simulink library "ddm"  (R2021b)
settings: Solver=VariableStepAuto  StartTime=0.0  StopTime=10.0  RelTol=1e-3
undefined symbols (not defined in the file): ADDM_FrTMTqDev_X_Nm, ADDM_RrTMTqDev_X_Nm, ENUM_ADASACCSTA_ERROR, ENUM_ADASACCSTA_OFF, ENUM_ADASACCSTA_STANDBY, ENUM_ALLOWMOV_ALLOWREADY, ENUM_APS, ENUM_BRKSTA_ERROR, ENUM_BRKSTA_OFF, ENUM_BRKSTA_ON, ENUM_BRKSW_INVALID, ENUM_BRKSW_OFF, ENUM_BRKSW_ON, ENUM_CHGPREACTERRSTA_OBCPRE, ENUM_DCDCFAULTSTA_ANYFAULTLV1, ENUM_DCDCFAULTSTA_ANYFAULTLV2, ENUM_DRIVETRAIN_AWD, ENUM_DRIVETRAIN_FWD, ENUM_DRIVETRAIN_RWD, ENUM_EDUDRTSTA_NORMAL, ENUM_EPBERROR_FAILED, ENUM_EPBSTA_APPLIED, ENUM_EPBSTA_RELEASED, ENUM_ESCAPSSta_APSUNAVAILABLE, ENUM_GEARACTUALPOSN_INVALID, ENUM_GEARACTUALPOSN_P, ENUM_HVBATTREADYPRE_READY, ENUM_HWRESETSTA_HWRESETING, ENUM_MCUWARN_LV0, ENUM_MCUWARN_LV1, ENUM_MCUWARN_LV2, ENUM_MCUWARN_LV3, ENUM_MCUWARN_NOERROR, ENUM_OBCFAULTSTA_ANYFAULT, ENUM_PAS_R2F2, ENUM_PDFAULT_BATTPDFAIL, ENUM_PDFAULT_DCDCDISABLE, ENUM_PDFAULT_MCUDISABLE, ENUM_PDFAULT_MCUDISCHRG, ENUM_POWERSTA_OFF, ENUM_POWERSTA_ON, ENUM_POWERSTA_READY, ENUM_POWERSTA_STANDBY, ENUM_PRESSINDI_LOW, ENUM_PUFAULT_BATTUPFAIL, ENUM_PUFAULT_DCDCENABLEFAIL, ENUM_PUFAULT_PRECHRGCHKFAIL, ENUM_PUFAULT_SAFETYCHKFAIL, ENUM_PWRSTASW_OFF, ENUM_PWRSTASW_OFFA, ENUM_PWRSTASW_OFFCHVCHRG, ENUM_PWRSTASW_OFFCLVCHRG, ENUM_PWRSTASW_ON, ENUM_PWRSTASW_ONHVCHRG, ENUM_PWRSTASW_READY, ENUM_PWRSTASW_STANDBY, ENUM_RAPSErrWarnSta_NORMAL, ENUM_RAPSErrWarnSta_RAPSERRLV1, ENUM_SHIFTCOMMAND_P, ENUM_SHIFTERERRSTA_PBUTTONFAILURE ... (+471)
libraries: hcu_lib x540, simulink x3
(part 6 of 26)

== system ddm/DDM/DDM/TPM ==
  note: SensorFail
  note: WheelTmpHigh
  note: PressureLow
  note: Batwarn
  task_time_s : Inport
  VPMM_PowerSta_enum : Inport  Port=2
  DTC_clear_request : Inport  Port=3
  VDDM_ClearZevDTCcmd_flg : Inport  Port=4
  VTPM_LFBatwarn_flg : Inport  Port=5
  VTPM_RFBatwarn_flg : Inport  Port=6
  VTPM_LRBatwarn_flg : Inport  Port=7
  VTPM_RRBatwarn_flg : Inport  Port=8
  VTPM_LFPressIndi_enum : Inport  Port=9
  VTPM_RFPressIndi_enum : Inport  Port=10
  VTPM_LRPressIndi_enum : Inport  Port=11
  VTPM_RRPressIndi_enum : Inport  Port=12
  VTPM_LFWheelTmpIndi_flg : Inport  Port=13
  VTPM_RFWheelTmpIndi_flg : Inport  Port=14
  VTPM_LRWheelTmpIndi_flg : Inport  Port=15
  VTPM_RRWheelTmpIndi_flg : Inport  Port=16
  VTPM_LFSensorFail_flg : Inport  Port=17
  VTPM_RFSensorFail_flg : Inport  Port=18
  VTPM_LRSensorFail_flg : Inport  Port=19
  VTPM_RRSensorFail_flg : Inport  Port=20
  LFBatwarn : Subsystem
  LFPressureLow : Subsystem
  LFSensorfail : Subsystem
  LFWheelTmpHigh : Subsystem
  LRBatwarn : Subsystem
  LRPressureLow : Subsystem
  LRSensorfail : Subsystem
  LRWheelTmpHigh : Subsystem
  RFBatwarn : Subsystem
  RFPressureLow : Subsystem
  RFSensorfail : Subsystem
  RFWheelTmpHigh : Subsystem
  RRBatwarn : Subsystem
  RRPressureLow : Subsystem
  RRSensorfail : Subsystem
  RRWheelTmpHigh : Subsystem
  VDDM_LFBatwarnDTC_raw32 : Outport
  VDDM_RFBatwarnDTC_raw32 : Outport  Port=2
  VDDM_LRBatwarnDTC_raw32 : Outport  Port=3
  VDDM_RRBatwarnDTC_raw32 : Outport  Port=4
  VDDM_LFPressIndiDTC_raw32 : Outport  Port=5
  VDDM_RFPressIndiDTC_raw32 : Outport  Port=6
  VDDM_LRPressIndiDTC_raw32 : Outport  Port=7
  VDDM_RRPressIndiDTC_raw32 : Outport  Port=8
  VDDM_LFWheelTmpHighDTC_raw32 : Outport  Port=9
  VDDM_RFWheelTmpHighDTC_raw32 : Outport  Port=10
  VDDM_LRWheelTmpHighDTC_raw32 : Outport  Port=11
  VDDM_RRWheelTmpHighDTC_raw32 : Outport  Port=12
  VDDM_LFSensorFailDTC_raw32 : Outport  Port=13
  VDDM_RFSensorFailDTC_raw32 : Outport  Port=14
  VDDM_LRSensorFailDTC_raw32 : Outport  Port=15
  VDDM_RRSensorFailDTC_raw32 : Outport  Port=16
  wires:
  VPMM_PowerSta_enum/1 -> [VPMM_PowerSta_enum]
  DTC_clear_request/1 -> [DTC_clear_request]
  task_time_s/1 -> [task_time_s]
  [VPMM_PowerSta_enum] -> LFBatwarn/2(VPMM_PowerSta_enum)
  [task_time_s] -> LFBatwarn/1(task_time_s)
  [DTC_clear_request] -> LFBatwarn/3(DTC_clear_request)
  VTPM_LFBatwarn_flg/1 -> LFBatwarn/4(VTPM_LFBatwarn_flg)
  LFBatwarn/1(VDDM_LFBatwarnDTC_raw32) -> VDDM_LFBatwarnDTC_raw32/1
  [task_time_s] -> RFBatwarn/1(task_time_s)
  [VPMM_PowerSta_enum] -> RFBatwarn/2(VPMM_PowerSta_enum)
  [DTC_clear_request] -> RFBatwarn/3(DTC_clear_request)
  VTPM_RFBatwarn_flg/1 -> RFBatwarn/4(VTPM_RFBatwarn_flg)
  RFBatwarn/1(VDDM_RFBatwarnDTC_raw32) -> VDDM_RFBatwarnDTC_raw32/1
  [task_time_s] -> LRBatwarn/1(task_time_s)
  [VPMM_PowerSta_enum] -> LRBatwarn/2(VPMM_PowerSta_enum)
  [DTC_clear_request] -> LRBatwarn/3(DTC_clear_request)
  VTPM_LRBatwarn_flg/1 -> LRBatwarn/4(VTPM_LRBatwarn_flg)
  LRBatwarn/1(VDDM_LRBatwarnDTC_raw32) -> VDDM_LRBatwarnDTC_raw32/1
  RRBatwarn/1(VDDM_RRBatwarnDTC_raw32) -> VDDM_RRBatwarnDTC_raw32/1
  [task_time_s] -> RRBatwarn/1(task_time_s)
  [VPMM_PowerSta_enum] -> RRBatwarn/2(VPMM_PowerSta_enum)
  [DTC_clear_request] -> RRBatwarn/3(DTC_clear_request)
  VTPM_RRBatwarn_flg/1 -> RRBatwarn/4(VTPM_RRBatwarn_flg)
  [task_time_s] -> LFPressureLow/1(task_time_s)
  [VPMM_PowerSta_enum] -> LFPressureLow/2(VPMM_PowerSta_enum)
  [VDDM_ClearZevDTCcmd_flg] -> LFPressureLow/3(DTC_clear_request)
  [task_time_s] -> RFPressureLow/1(task_time_s)
  [VPMM_PowerSta_enum] -> RFPressureLow/2(VPMM_PowerSta_enum)
  [VDDM_ClearZevDTCcmd_flg] -> RFPressureLow/3(DTC_clear_request)
  [VDDM_ClearZevDTCcmd_flg] -> LRPressureLow/3(DTC_clear_request)
  [VPMM_PowerSta_enum] -> LRPressureLow/2(VPMM_PowerSta_enum)
  [task_time_s] -> LRPressureLow/1(task_time_s)
  [task_time_s] -> RRPressureLow/1(task_time_s)
  [VPMM_PowerSta_enum] -> RRPressureLow/2(VPMM_PowerSta_enum)
  [VDDM_ClearZevDTCcmd_flg] -> RRPressureLow/3(DTC_clear_request)
  LFPressureLow/1(VDDM_LFPressIndiDTC_raw32) -> VDDM_LFPressIndiDTC_raw32/1
  RFPressureLow/1(VDDM_RFPressIndiDTC_raw32) -> VDDM_RFPressIndiDTC_raw32/1
  LRPressureLow/1(VDDM_LRPressIndiDTC_raw32) -> VDDM_LRPressIndiDTC_raw32/1
  RRPressureLow/1(VDDM_RRPressIndiDTC_raw32) -> VDDM_RRPressIndiDTC_raw32/1
  VTPM_LFPressIndi_enum/1 -> LFPressureLow/4(VTPM_LFPressIndi_enum)
  VTPM_RFPressIndi_enum/1 -> RFPressureLow/4(VTPM_RFPressIndi_enum)
  VTPM_LRPressIndi_enum/1 -> LRPressureLow/4(VTPM_LRPressIndi_enum)
  VTPM_RRPressIndi_enum/1 -> RRPressureLow/4(VTPM_RRPressIndi_enum)
  [task_time_s] -> LFWheelTmpHigh/1(task_time_s)
  [VPMM_PowerSta_enum] -> LFWheelTmpHigh/2(VPMM_PowerSta_enum)
  [DTC_clear_request] -> LFWheelTmpHigh/3(DTC_clear_request)
  [task_time_s] -> RFWheelTmpHigh/1(task_time_s)
  [VPMM_PowerSta_enum] -> RFWheelTmpHigh/2(VPMM_PowerSta_enum)
  [DTC_clear_request] -> RFWheelTmpHigh/3(DTC_clear_request)
  [task_time_s] -> LRWheelTmpHigh/1(task_time_s)
  [VPMM_PowerSta_enum] -> LRWheelTmpHigh/2(VPMM_PowerSta_enum)
  [DTC_clear_request] -> LRWheelTmpHigh/3(DTC_clear_request)
  [task_time_s] -> RRWheelTmpHigh/1(task_time_s)
  [VPMM_PowerSta_enum] -> RRWheelTmpHigh/2(VPMM_PowerSta_enum)
  [DTC_clear_request] -> RRWheelTmpHigh/3(DTC_clear_request)
  VTPM_LFWheelTmpIndi_flg/1 -> LFWheelTmpHigh/4(VTPM_LFWheelTmpHigh_flg)
  VTPM_RFWheelTmpIndi_flg/1 -> RFWheelTmpHigh/4(VTPM_RFWheelTmpHigh_flg)
  VTPM_LRWheelTmpIndi_flg/1 -> LRWheelTmpHigh/4(VTPM_LRWheelTmpHigh_flg)
  VTPM_RRWheelTmpIndi_flg/1 -> RRWheelTmpHigh/4(VTPM_RRWheelTmpHigh_flg)
  LFWheelTmpHigh/1(VDDM_LFWheelTmpHighDTC_raw32) -> VDDM_LFWheelTmpHighDTC_raw32/1
  RFWheelTmpHigh/1(VDDM_RFWheelTmpHighDTC_raw32) -> VDDM_RFWheelTmpHighDTC_raw32/1
  LRWheelTmpHigh/1(VDDM_LRWheelTmpHighDTC_raw32) -> VDDM_LRWheelTmpHighDTC_raw32/1
  RRWheelTmpHigh/1(VDDM_RRWheelTmpHighDTC_raw32) -> VDDM_RRWheelTmpHighDTC_raw32/1
  [task_time_s] -> LFSensorfail/1(task_time_s)
  [VPMM_PowerSta_enum] -> LFSensorfail/2(VPMM_PowerSta_enum)
  [VDDM_ClearZevDTCcmd_flg] -> LFSensorfail/3(DTC_clear_request)
  [task_time_s] -> RFSensorfail/1(task_time_s)
  [VPMM_PowerSta_enum] -> RFSensorfail/2(VPMM_PowerSta_enum)
  [VDDM_ClearZevDTCcmd_flg] -> RFSensorfail/3(DTC_clear_request)
  [task_time_s] -> LRSensorfail/1(task_time_s)
  [VPMM_PowerSta_enum] -> LRSensorfail/2(VPMM_PowerSta_enum)
  [VDDM_ClearZevDTCcmd_flg] -> LRSensorfail/3(DTC_clear_request)
  [task_time_s] -> RRSensorfail/1(task_time_s)
  [VPMM_PowerSta_enum] -> RRSensorfail/2(VPMM_PowerSta_enum)
  [VDDM_ClearZevDTCcmd_flg] -> RRSensorfail/3(DTC_clear_request)
  VTPM_LFSensorFail_flg/1 -> LFSensorfail/4(VTPM_LFSensorFail_flg)
  VTPM_RFSensorFail_flg/1 -> RFSensorfail/4(VTPM_RFSensorFail_flg)
  VTPM_LRSensorFail_flg/1 -> LRSensorfail/4(VTPM_LRSensorFail_flg)
  VTPM_RRSensorFail_flg/1 -> RRSensorfail/4(VTPM_RRSensorFail_flg)
  LFSensorfail/1(VDDM_LFSensorFailDTC_raw32) -> VDDM_LFSensorFailDTC_raw32/1
  RFSensorfail/1(VDDM_RFSensorFailDTC_raw32) -> VDDM_RFSensorFailDTC_raw32/1
  LRSensorfail/1(VDDM_LRSensorFailDTC_raw32) -> VDDM_LRSensorFailDTC_raw32/1
  RRSensorfail/1(VDDM_RRSensorFailDTC_raw32) -> VDDM_RRSensorFailDTC_raw32/1
  VDDM_ClearZevDTCcmd_flg/1 -> [VDDM_ClearZevDTCcmd_flg]

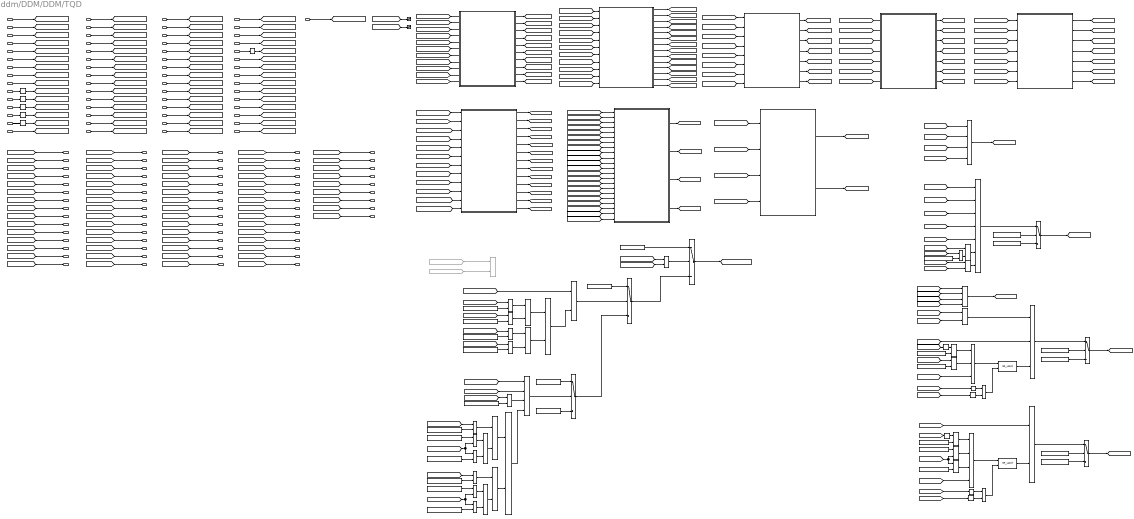
== system ddm/DDM/DDM/TQD ==
  note: VDDM_EPB1Err_flg
  note: Shifeter Error lamp Signal
  note: Three-electrical warning
  note: Warning lamp Signal
  note: RAPS Signal error
  VPMM_SysPwrSta_enum : Inport
  VINP_AccelPedal1Vol_V : Inport  Port=2
  VINP_AccelPedal2Vol_V : Inport  Port=3
  VDHP_EAPS12RangeSta_enum : Inport  Port=4
  VDHP_EAPCRBAD_flg : Inport  Port=5
  task_time_s : Inport  Port=6
  DTC_clear_request : Inport  Port=7
  No_CAN3_BUS_OFF : Inport  Port=8
  No_CAN1_BUS_OFF : Inport  Port=9
  VDDM_CANMsgValidMCUF1_flg : Inport  Port=10
  VDDM_CANMsgValidMCUR1_flg : Inport  Port=11
  VINP_CANMsgValidShifter1_flg : Inport  Port=12
  VINP_CANMsgValidESC1_flg : Inport  Port=13
  VINP_CANMsgValidESC5_flg : Inport  Port=14
  VDDM_MCUF1RCErr_flg : Inport  Port=15
  VDDM_MCUF1CSErr_flg : Inport  Port=16
  VDDM_MCUR1RCErr_flg : Inport  Port=17
  VDDM_MCUR1CSErr_flg : Inport  Port=18
  VDDM_Shifter1RCErr_flg : Inport  Port=19
  VDDM_Shifter1CSErr_flg : Inport  Port=20
  VDDM_ESC1RCErr_flg : Inport  Port=21
  VDDM_ESC1CSErr_flg : Inport  Port=22
  VDDM_ESC5RCErr_flg : Inport  Port=23
  VDDM_ESC5CSErr_flg : Inport  Port=24
  VINP_FrEDUDrtSta_flg : Inport  Port=25
  VINP_VehSpeed_kph : Inport  Port=26
  VINP_FrEDURealTMTq_Nm : Inport  Port=27
  VTQR_FrTMTqReq_Nm : Inport  Port=28
  VINP_RrEDUDrtSta_flg : Inport  Port=29
  VINP_RrEDURealTMTq_Nm : Inport  Port=30
  VTQR_RrTMTqReq_Nm : Inport  Port=31
  VINP_MCUWarnF_enum : Inport  Port=32
  VINP_MCUWarnR_enum : Inport  Port=33
  VINP_Pedal1Ref5V_V : Inport  Port=34
  VINP_Pedal2Ref5V_V : Inport  Port=35
  VINP_HVBattSOC_pct : Inport  Port=36
  VDDM_AuxBattVolV_V : Inport  Port=37
  VTQD_ActParkRequest_flg : Inport  Port=38
  VINP_EPBSta_enum : Inport  Port=39
  VINP_ShifterHandleCmd_enum : Inport  Port=40
  VINP_BMSWarn4_flg : Inport  Port=41
  VINP_BMSWarn5_flg : Inport  Port=42
  VINP_BMSWarn6_flg : Inport  Port=43
  VINP_BMSWarn7_flg : Inport  Port=44
  VINP_BMSWarn8_flg : Inport  Port=45
  VINP_DCDCFaultSta_enum : Inport  Port=46
  VPMM_DrivetrainSelect_enum : Inport  Port=47
  VTQD_GearActualPosn_enum : Inport  Port=48
  VINP_EPBErrSta_enum : Inport  Port=49
  VINP_CANMsgValidEPB1_flg : Inport  Port=50
  VDDM_EPB1RCErr_flg : Inport  Port=51
  VDDM_EPB1CSErr_flg : Inport  Port=52
  VDHP_EAPS1BAD_flg : Inport  Port=53
  VDHP_EAPS2BAD_flg : Inport  Port=54
  VDDM_C3BMS1LCCFS_flg : Inport  Port=55
  VDDM_VCURAPSErrLv2_flg : Inport  Port=56
  VVMC_APSActive_flg : Inport  Port=57
  VDDM_ClearZevDTCcmd_flg : Inport  Port=58
  VDDM_LimpHomeAct_flg : Inport  Port=59
  VTQR_FrTqZeroTrans_enum : Inport  Port=60
  VTQR_RrTqZeroTrans_enum : Inport  Port=61
  APS_DDM : Subsystem
  Constant : Constant  Value=KDDM_SysErrShifterErrSW_flg
  Constant1 : Constant  Value=ENUM_DRIVETRAIN_FWD
  Constant10 : Constant  Value=ENUM_MCUWARN_LV3
  Constant11 : Constant  Value=ENUM_VEHMALFUNLV_3RD
  Constant12 : Constant  Value=ENUM_VEHMALFUNLV_4TH
  Constant{13..14,18..19,88} (5 alike) : Constant  Value=ENUM_GEARACTUALPOSN_P
  Constant15 : Constant  Value=ENUM_VEHMALFUNLV_2ND
  Constant16 : Constant  Value=ENUM_VEHMALFUNLV_NORMAL
  Constant17 : Constant  Value=ENUM_DCDCFAULTSTA_ANYFAULTLV2
  Constant2 : Constant  Value=ENUM_MCUWARN_LV1
  Constant20 : Constant  Value=ENUM_GEARACTUALPOSN_INVALID
  Constant21 : Constant  Value=FALSE
  Constant22 : Constant  Value=KDDM_EPBErrPopupSW_flg
  Constant23 : Constant  Value=FALSE
  Constant24 : Constant  Value=KDDM_EPBErrPopupSW_flg
  Constant25 : Constant  Value=FALSE
  Constant3 : Constant  Value=ENUM_MCUWARN_LV2
  Constant4 : Constant  Value=ENUM_DRIVETRAIN_RWD
  Constant5 : Constant  Value=ENUM_MCUWARN_LV1
  Constant6 : Constant  Value=ENUM_MCUWARN_LV2
  Constant7 : Constant  Value=ENUM_DRIVETRAIN_FWD
  Constant8 : Constant  Value=ENUM_DRIVETRAIN_RWD
  Constant9 : Constant  Value=ENUM_MCUWARN_LV3
  Delay{,1..3} (4 alike) : Delay  DelayLength=1
  EPB : Subsystem
  ESC1_DDM : Subsystem
  ESC5_DDM : Subsystem
  Equal{,1,5,8,11,15..16} (7 alike) : RelationalOperator  Operator=~=  OutDataTypeStr=boolean  RndMeth=Simplest
  Equal{2..4,6..7,9..10,12..14} (10 alike) : RelationalOperator  Operator===  OutDataTypeStr=boolean  RndMeth=Simplest
  From112 : From  Commented=on  GotoTag=VDDM_MCUNR1NoComCFS_flg
  From176 : From  Commented=on  GotoTag=VDDM_C3BMS1LCCFS_flg
  Logical Operator{,1,3..5,8,12..13} (8 alike) : Logic  Operator=NOT  AllPortsSameDT=off  OutDataTypeStr=boolean
  Logical Operator10 : Logic  Inputs=4  AllPortsSameDT=off  OutDataTypeStr=boolean
  Logical Operator11 : Logic  AllPortsSameDT=off  OutDataTypeStr=boolean
  Logical Operator14 : Logic  Operator=OR  AllPortsSameDT=off  OutDataTypeStr=boolean
  Logical Operator15 : Logic  Operator=OR  AllPortsSameDT=off  OutDataTypeStr=boolean
  Logical Operator2 : Logic  AllPortsSameDT=off  OutDataTypeStr=boolean
  Logical Operator6 : Logic  AllPortsSameDT=off  OutDataTypeStr=boolean
  Logical Operator7 : Logic  Inputs=3  AllPortsSameDT=off  OutDataTypeStr=boolean
  Logical Operator9 : Logic  Operator=OR  Inputs=4  AllPortsSameDT=off  OutDataTypeStr=boolean
  MCU1_DDM : Subsystem
  MCU_DDM : Subsystem
  OR : Logic  Operator=OR  Inputs=4  AllPortsSameDT=off  OutDataTypeStr=boolean
  OR1 : Logic  Operator=OR  Inputs=7  AllPortsSameDT=off  OutDataTypeStr=boolean
  OR{4,6..7,9..10,12,14} (7 alike) : Logic  Operator=OR  AllPortsSameDT=off  OutDataTypeStr=boolean
  OR{5,8,11,13} (4 alike) : Logic  AllPortsSameDT=off  OutDataTypeStr=boolean
  OR15 : Logic  Commented=on  Operator=OR  AllPortsSameDT=off  OutDataTypeStr=boolean
  OR2 : Logic  Operator=OR  Inputs=3  AllPortsSameDT=off  OutDataTypeStr=boolean
  OR3 : Logic  Operator=OR  Inputs=4  AllPortsSameDT=off  OutDataTypeStr=boolean
  Regen_fail_DDM : Subsystem
  SR_Latch1 : hcu_lib/Basic_Blocks/SR_Latch
  SR_Latch2 : hcu_lib/Basic_Blocks/SR_Latch
  Shifter1_DDM : Subsystem
  Switch : Switch  Criteria=u2 > Threshold
  Switch1 : Switch  Criteria=u2 ~= 0
  Switch2 : Switch  Criteria=u2 ~= 0
  Switch3 : Switch  Criteria=u2 > Threshold
  Switch4 : Switch  Criteria=u2 > Threshold
  Switch6 : Switch  Criteria=u2 ~= 0
  Terminator : Terminator
  Terminator1 : Terminator
  VDDM_APS1SigOoRDTC_raw32 : Outport
  VDDM_APS2SigOoRDTC_raw32 : Outport  Port=2
  VDDM_APSCorrErrDTC_raw32 : Outport  Port=3
  VDDM_MCUF1NoComDTC_raw32 : Outport  Port=4
  VDDM_MCUR1NoComDTC_raw32 : Outport  Port=5
  VDDM_Shifter1NoComDTC_raw32 : Outport  Port=6
  VDDM_ESC1NoComDTC_raw32 : Outport  Port=7
  VDDM_ESC5NoComDTC_raw32 : Outport  Port=8
  VDDM_MCUF1RCErrDTC_raw32 : Outport  Port=9
  VDDM_MCUR1RCErrDTC_raw32 : Outport  Port=10
  VDDM_MCUF1CSErrDTC_raw32 : Outport  Port=11
  VDDM_MCUR1CSErrDTC_raw32 : Outport  Port=12
  VDDM_Shifter1RCErrDTC_raw32 : Outport  Port=13
  VDDM_Shifter1CSErrDTC_raw32 : Outport  Port=14
  VDDM_ESC1RCErrDTC_raw32 : Outport  Port=15
  VDDM_ESC1CSErrDTC_raw32 : Outport  Port=16
  VDDM_ESC5RCErrDTC_raw32 : Outport  Port=17
  VDDM_ESC5CSErrDTC_raw32 : Outport  Port=18
  VDDM_FrMCUTqErrDTC_raw32 : Outport  Port=19
  VDDM_RrMCUTqErrDTC_raw32 : Outport  Port=20
  VDDM_MCUF1NoComCFS_flg : Outport  Port=21
  VDDM_MCUF1RCErrCFS_flg : Outport  Port=22
  VDDM_MCUF1CSErrCFS_flg : Outport  Port=23
  VDDM_MCUR1NoComCFS_flg : Outport  Port=24
  VDDM_MCUR1RCErrCFS_flg : Outport  Port=25
  VDDM_MCUR1CSErrCFS_flg : Outport  Port=26
  VDDM_ESC1NoComCFS_flg : Outport  Port=27
  VDDM_ESC1RCErrCFS_flg : Outport  Port=28
  VDDM_ESC1CSErrCFS_flg : Outport  Port=29
  VDDM_ESC5NoComCFS_flg : Outport  Port=30
  VDDM_ESC5RCErrCFS_flg : Outport  Port=31
  VDDM_ESC5CSErrCFS_flg : Outport  Port=32
  VDDM_5vAPS1OoRDTC_raw32 : Outport  Port=33
  VDDM_5vAPS2OoRDTC_raw32 : Outport  Port=34
  VDDM_EDriveSysErrTQD_flg : Outport  Port=35
  VDDM_EDriveSysErrShifterErr_flg : Outport  Port=36
  VDDM_EngagePFail_flg : Outport  Port=37
  VDDM_VehMalfunLevelTmp_enum : Outport  Port=38
  VDDM_EPBLockTODTC_raw32 : Outport  Port=39
  VDDM_EPBUnlockTODTC_raw32 : Outport  Port=40
  VDDM_EPB1NoComDTC_raw32 : Outport  Port=41
  VDDM_EPB1RCErrDTC_raw32 : Outport  Port=42
  VDDM_EPB1CSErrDTC_raw32 : Outport  Port=43
  VDDM_EPBSigErrDTC_raw32 : Outport  Port=44
  VDDM_5vAPS1OoRCFS_flg : Outport  Port=45
  VDDM_5vAPS2OoRCFS_flg : Outport  Port=46
  VDDM_APS1SigOoRCFS_flg : Outport  Port=47
  VDDM_APS2SigOoRCFS_flg : Outport  Port=48
  VDDM_APSCorrErrCFS_flg : Outport  Port=49
  VDDM_Shifter1NoComCFS_flg : Outport  Port=50
  VDDM_Shifter1RCErrCFS_flg : Outport  Port=51
  VDDM_Shifter1CSErrCFS_flg : Outport  Port=52
  VDDM_EPBSigErrCFS_flg : Outport  Port=53
  VDDM_EPB1NoComCFS_flg : Outport  Port=54
  VDDM_EPB1RCErrCFS_flg : Outport  Port=55
  VDDM_EPB1CSErrCFS_flg : Outport  Port=56
  VDDM_EPBLockTOCFS_flg : Outport  Port=57
  VDDM_EPBUnlockTOCFS_flg : Outport  Port=58
  VDDM_FrMCUTqErrCFS_flg : Outport  Port=59
  VDDM_RrMCUTqErrCFS_flg : Outport  Port=60
  VDDM_DisengagePFail_flg : Outport  Port=61
  VDDM_Shifter1Err_flg : Outport  Port=62
  VDDM_EPB1Err_flg : Outport  Port=63
  VDDM_ESC5Err_flg : Outport  Port=64
  VDDM_ESC1Err_flg : Outport  Port=65
  VDDM_RegenErrDTC_raw32 : Outport  Port=66
  VDDM_RegenErrCFS_flg : Outport  Port=67
  VDDM_MCUF1Err_flg : Outport  Port=68
  VDDM_MCUR1Err_flg : Outport  Port=69
  wires:
  VINP_ShifterHandleCmd_enum/1 -> [VINP_ShifterHandleCmd_enum]
  VINP_EPBSta_enum/1 -> [VINP_EPBSta_enum]
  VTQD_ActParkRequest_flg/1 -> [VTQD_ActParkRequest_flg]
  VDDM_AuxBattVolV_V/1 -> [VDDM_AuxBattVolV_V]
  VINP_HVBattSOC_pct/1 -> [VINP_HVBattSOC_pct]
  [VINP_Pedal2Ref5V_V] -> APS_DDM/7(VINP_Pedal2Ref5V_V)
  [VINP_Pedal1Ref5V_V] -> APS_DDM/6(VINP_Pedal1Ref5V_V)
  VINP_Pedal2Ref5V_V/1 -> [VINP_Pedal2Ref5V_V]
  VINP_Pedal1Ref5V_V/1 -> [VINP_Pedal1Ref5V_V]
  [VDDM_MCUR1RCErrCFS_flg] -> MCU_DDM/12(VDDM_MCUR1RCErrCFS_flg)
  [VDDM_MCUF1RCErrCFS_flg] -> MCU_DDM/5(VDDM_MCUF1RCErrCFS_flg)
  [VDDM_MCUF1CSErrCFS_flg] -> MCU_DDM/6(VDDM_MCUF1CSErrCFS_flg)
  [No_CAN3_BUS_OFF] -> MCU_DDM/3(No_CAN3_BUS_OFF)
  [VINP_MCUWarnF_enum] -> MCU_DDM/17(VINP_MCUWarnF_enum)
  [VINP_RrEDUDrtSta_flg] -> MCU_DDM/14(VINP_RrEDUDrtSta_flg)
  [VDDM_MCUR1CSErrCFS_flg] -> MCU_DDM/13(VDDM_MCUR1CSErrCFS_flg)
  [VPMM_SysPwrSta_enum] -> MCU_DDM/2(VPMM_SysPwrSta_enum)
  [VDDM_MCUF1NoComCFS_flg] -> MCU_DDM/4(VDDM_MCUF1NoComCFS_flg)
  [VTQR_FrTMTqReq_Nm] -> MCU_DDM/10(VTQR_FrTMTqReq_Nm)
  [task_time_s] -> MCU_DDM/1(task_time_s)
  [VTQR_RrTMTqReq_Nm] -> MCU_DDM/16(VTQR_RrTMTqReq_Nm)
  [VINP_FrEDUDrtSta_flg] -> MCU_DDM/8(VINP_FrEDUDrtSta_flg)
  [VINP_FrEDURealTMTq_Nm] -> MCU_DDM/9(VINP_FrEDURealTMTq_Nm)
  [VINP_RrEDURealTMTq_Nm] -> MCU_DDM/15(VINP_RrEDURealTMTq_Nm)
  [VDDM_ClearZevDTCcmd_flg] -> MCU_DDM/19(DTC_clear_request)
  [VDDM_MCUR1NoComCFS_flg] -> MCU_DDM/11(VDDM_MCUR1NoComCFS_flg)
  [VINP_MCUWarnR_enum] -> MCU_DDM/18(VINP_MCUWarnR_enum)
  [VINP_VehSpeed_kph] -> MCU_DDM/7(VINP_VehSpeed_kph)
  [VDDM_MCUF1RCErrCFS_flg] -> VDDM_MCUF1RCErrCFS_flg/1
  [VDDM_MCUR1RCErrCFS_flg] -> VDDM_MCUR1RCErrCFS_flg/1
  [VDDM_MCUR1NoComCFS_flg] -> VDDM_MCUR1NoComCFS_flg/1
  [VDDM_MCUF1CSErrCFS_flg] -> VDDM_MCUF1CSErrCFS_flg/1
  [VDDM_MCUR1CSErrCFS_flg] -> VDDM_MCUR1CSErrCFS_flg/1
  [VDDM_MCUF1NoComCFS_flg] -> VDDM_MCUF1NoComCFS_flg/1
  MCU1_DDM/11(VDDM_MCUR1RCErrCFS_flg) -> [VDDM_MCUR1RCErrCFS_flg]
  MCU1_DDM/7(VDDM_MCUF1NoComCFS_flg) -> [VDDM_MCUF1NoComCFS_flg]
  MCU1_DDM/10(VDDM_MCUR1NoComCFS_flg) -> [VDDM_MCUR1NoComCFS_flg]
  MCU1_DDM/9(VDDM_MCUF1CSErrCFS_flg) -> [VDDM_MCUF1CSErrCFS_flg]
  MCU1_DDM/8(VDDM_MCUF1RCErrCFS_flg) -> [VDDM_MCUF1RCErrCFS_flg]
  MCU1_DDM/12(VDDM_MCUR1CSErrCFS_flg) -> [VDDM_MCUR1CSErrCFS_flg]
  VINP_MCUWarnR_enum/1 -> [VINP_MCUWarnR_enum]
  VINP_MCUWarnF_enum/1 -> [VINP_MCUWarnF_enum]
  VINP_VehSpeed_kph/1 -> [VINP_VehSpeed_kph]
  VINP_RrEDUDrtSta_flg/1 -> [VINP_RrEDUDrtSta_flg]
  VTQR_FrTMTqReq_Nm/1 -> [VTQR_FrTMTqReq_Nm]
  VINP_FrEDURealTMTq_Nm/1 -> [VINP_FrEDURealTMTq_Nm]
  VTQR_RrTMTqReq_Nm/1 -> [VTQR_RrTMTqReq_Nm]
  VINP_FrEDUDrtSta_flg/1 -> [VINP_FrEDUDrtSta_flg]
  VINP_RrEDURealTMTq_Nm/1 -> [VINP_RrEDURealTMTq_Nm]
  VDDM_ESC5RCErr_flg/1 -> [VDDM_ESC5RCErr_flg]
  VDDM_ESC5CSErr_flg/1 -> [VDDM_ESC5CSErr_flg]
  [VDDM_ESC5CSErr_flg] -> ESC5_DDM/6(VDDM_ESC5CSErr_flg)
  [VDDM_ESC5RCErr_flg] -> ESC5_DDM/5(VDDM_ESC5RCErr_flg)
  VDDM_ESC1RCErr_flg/1 -> [VDDM_ESC1RCErr_flg]
  VDDM_ESC1CSErr_flg/1 -> [VDDM_ESC1CSErr_flg]
  VDDM_Shifter1CSErr_flg/1 -> [VDDM_Shifter1CSErr_flg]
  VDDM_Shifter1RCErr_flg/1 -> [VDDM_Shifter1RCErr_flg]
  VDDM_MCUF1RCErr_flg/1 -> [VDDM_MCUF1RCErr_flg]
  VDDM_MCUF1CSErr_flg/1 -> [VDDM_MCUF1CSErr_flg]
  VDDM_MCUR1CSErr_flg/1 -> [VDDM_MCUR1CSErr_flg]
  VDDM_MCUR1RCErr_flg/1 -> [VDDM_MCUR1RCErr_flg]
  [VDDM_Shifter1CSErr_flg] -> Shifter1_DDM/6(VDDM_Shifter1CSErr_flg)
  [VDDM_Shifter1RCErr_flg] -> Shifter1_DDM/5(VDDM_Shifter1RCErr_flg)
  [VDDM_MCUR1CSErr_flg] -> MCU1_DDM/9(VDDM_MCUR1CSErr_flg)
  [VDDM_MCUR1RCErr_flg] -> MCU1_DDM/8(VDDM_MCUR1RCErr_flg)
  [VDDM_MCUF1CSErr_flg] -> MCU1_DDM/7(VDDM_MCUF1CSErr_flg)
  [VDDM_MCUF1RCErr_flg] -> MCU1_DDM/6(VDDM_MCUF1RCErr_flg)
  Logical Operator5/1 -> [VDDM_MCUF1NoCom_flg]
  Logical Operator4/1 -> [VDDM_MCUR1NoCom_flg]
  Logical Operator3/1 -> [VDDM_Shifter1NoCom_flg]
  Logical Operator1/1 -> [VDDM_ESC1NoCom_flg]
  Logical Operator/1 -> [VDDM_ESC5NoCom_flg]
  VINP_CANMsgValidESC5_flg/1 -> Logical Operator/1
  VINP_CANMsgValidESC1_flg/1 -> Logical Operator1/1
  VINP_CANMsgValidShifter1_flg/1 -> Logical Operator3/1
  VDDM_CANMsgValidMCUR1_flg/1 -> Logical Operator4/1
  VDDM_CANMsgValidMCUF1_flg/1 -> Logical Operator5/1
  No_CAN1_BUS_OFF/1 -> [No_CAN1_BUS_OFF]
  No_CAN3_BUS_OFF/1 -> [No_CAN3_BUS_OFF]
  [VDDM_ClearZevDTCcmd_flg] -> ESC5_DDM/7(DTC_clear_request)
  [VDDM_ESC5NoCom_flg] -> ESC5_DDM/4(VDDM_ESC5NoCom_flg)
  [No_CAN1_BUS_OFF] -> ESC5_DDM/3(No_CAN1_BUS_OFF)
  [VPMM_SysPwrSta_enum] -> ESC5_DDM/2(VPMM_SysPwrSta_enum)
  [task_time_s] -> ESC5_DDM/1(task_time_s)
  [No_CAN1_BUS_OFF] -> ESC1_DDM/3(No_CAN1_BUS_OFF)
  [VPMM_SysPwrSta_enum] -> ESC1_DDM/2(VPMM_SysPwrSta_enum)
  [task_time_s] -> ESC1_DDM/1(task_time_s)
  [VDDM_ClearZevDTCcmd_flg] -> Shifter1_DDM/7(DTC_clear_request)
  [VDDM_Shifter1NoCom_flg] -> Shifter1_DDM/4(VDDM_Shifter1NoCom_flg)
  [No_CAN3_BUS_OFF] -> Shifter1_DDM/3(No_CAN3_BUS_OFF)
  [VPMM_SysPwrSta_enum] -> Shifter1_DDM/2(VPMM_SysPwrSta_enum)
  [VDDM_ClearZevDTCcmd_flg] -> MCU1_DDM/10(DTC_clear_request)
  [VDDM_MCUR1NoCom_flg] -> MCU1_DDM/5(VDDM_MCUR1NoCom_flg)
  [VDDM_MCUF1NoCom_flg] -> MCU1_DDM/4(VDDM_MCUF1NoCom_flg)
  [No_CAN3_BUS_OFF] -> MCU1_DDM/3(No_CAN3_BUS_OFF)
  [VPMM_SysPwrSta_enum] -> MCU1_DDM/2(VPMM_SysPwrSta_enum)
  [task_time_s] -> Shifter1_DDM/1(task_time_s)
  [task_time_s] -> MCU1_DDM/1(task_time_s)
  DTC_clear_request/1 -> [DTC_clear_request]
  task_time_s/1 -> [task_time_s]
  [VDHP_EAPS12RangeSta_enum] -> APS_DDM/4(VDHP_EAPS12RangeSta_enum)
  [VINP_AccelPedal2Vol_V] -> APS_DDM/3(VINP_AccelPedal2Vol_V)
  [VINP_AccelPedal1Vol_V] -> APS_DDM/2(VINP_AccelPedal1Vol_V)
  [VPMM_SysPwrSta_enum] -> APS_DDM/1(VPMM_SysPwrSta_enum)
  [VDHP_EAPCRBAD_flg] -> APS_DDM/5(VDHP_EAPCRBAD_flg)
  VPMM_SysPwrSta_enum/1 -> [VPMM_SysPwrSta_enum]
  VINP_AccelPedal1Vol_V/1 -> [VINP_AccelPedal1Vol_V]
  VDHP_EAPCRBAD_flg/1 -> [VDHP_EAPCRBAD_flg]
  VDHP_EAPS12RangeSta_enum/1 -> [VDHP_EAPS12RangeSta_enum]
  VINP_AccelPedal2Vol_V/1 -> [VINP_AccelPedal2Vol_V]
  Shifter1_DDM/4(VDDM_Shifter1NoComCFS_flg) -> [VDDM_Shifter1NoComCFS_flg]
  Shifter1_DDM/5(VDDM_Shifter1RCErrCFS_flg) -> [VDDM_Shifter1RCErrCFS_flg]
  Shifter1_DDM/6(VDDM_Shifter1CSErrCFS_flg) -> [VDDM_Shifter1CSErrCFS_flg]
  Switch/1 -> [VDDM_EDriveSysErrShifterErr_flg]  "VDDM_EDriveSysErrShifterErr_flg"
  [VDDM_Shifter1RCErrCFS_flg] -> OR1/2
  [VDDM_Shifter1NoComCFS_flg] -> OR1/1
  [VDDM_Shifter1CSErrCFS_flg] -> OR1/3
  [VDDM_EPBLockTOCFS_flg] -> OR1/4
  [VDDM_EPBUnlockTOCFS_flg] -> OR1/5
  [VDDM_Shifter1RCErrCFS_flg] -> OR/2
  [VDDM_Shifter1CSErrCFS_flg] -> OR/3
  [VDDM_Shifter1NoComCFS_flg] -> OR/1
  VINP_BMSWarn4_flg/1 -> [VINP_BMSWarn4_flg]
  VINP_BMSWarn5_flg/1 -> [VINP_BMSWarn5_flg]
  VINP_BMSWarn6_flg/1 -> [VINP_BMSWarn6_flg]
  VINP_BMSWarn7_flg/1 -> [VINP_BMSWarn7_flg]
  VINP_BMSWarn8_flg/1 -> [VINP_BMSWarn8_flg]
  VINP_DCDCFaultSta_enum/1 -> [VINP_DCDCFaultSta_enum]
  VPMM_DrivetrainSelect_enum/1 -> [VPMM_DrivetrainSelect_enum]
  [VDDM_VehMalfunLevelTmp_enum] -> VDDM_VehMalfunLevelTmp_enum/1
  [VPMM_DrivetrainSelect_enum] -> MCU1_DDM/11(VPMM_DrivetrainSelect_enum)
  [VINP_ShifterHandleCmd_enum] -> Shifter1_DDM/8(VINP_ShifterHandleCmd_enum)
  VTQD_GearActualPosn_enum/1 -> [VTQD_GearActualPosn_enum]
  [VDDM_ESC1NoCom_flg] -> ESC1_DDM/4(VDDM_ESC1NoCom_flg)
  [VDDM_ESC1RCErr_flg] -> ESC1_DDM/5(VDDM_ESC1RCErr_flg)
  [VDDM_ESC1CSErr_flg] -> ESC1_DDM/6(VDDM_ESC1CSErr_flg)
  [VDDM_ClearZevDTCcmd_flg] -> ESC1_DDM/7(DTC_clear_request)
  [VTQD_ActParkRequest_flg] -> EPB/5(VTQD_ActParkRequest_flg)
  EPB/10(VDDM_EPB1NoComCFS_flg) -> [VDDM_EPB1NoComCFS_flg]
  [VDDM_ClearZevDTCcmd_flg] -> EPB/9(DTC_clear_request)
  [No_CAN1_BUS_OFF] -> EPB/1(NO_CAN1_BUS_OFF)
  [VDDM_EPB1NoCom_flg] -> EPB/10(VDDM_EPB1NoCom_flg)
  [task_time_s] -> EPB/8(task_time_s)
  [VPMM_SysPwrSta_enum] -> EPB/4(VPMM_SysPwrSta_enum)
  EPB/3(VDDM_EPBLockTOCFS_flg) -> [VDDM_EPBLockTOCFS_flg]
  EPB/4(VDDM_EPBUnlockTOCFS_flg) -> [VDDM_EPBUnlockTOCFS_flg]
  EPB/9(VDDM_EPBSigErrCFS_flg) -> [VDDM_EPBSigErrCFS_flg]
  EPB/11(VDDM_EPB1RCErrCFS_flg) -> [VDDM_EPB1RCErrCFS_flg]
  [VINP_EPBSta_enum] -> EPB/6(VINP_EPBSta_enum)
  [VTQD_GearActualPosn_enum] -> EPB/2(VTQD_GearActualPosn_enum)
  [VDDM_EPB1RCErr_flg] -> EPB/11(VDDM_EPB1RCErr_flg)
  [VINP_EPBErrSta_enum] -> EPB/3(VINP_EPBErrSta_enum)
  [VDDM_EPB1CSErr_flg] -> EPB/12(VDDM_EPB1CSErr_flg)
  EPB/12(VDDM_EPB1CSErrCFS_flg) -> [VDDM_EPB1CSErrCFS_flg]
  [VINP_ShifterHandleCmd_enum] -> EPB/7(VINP_ShifterHandleCmd_enum)
  VINP_EPBErrSta_enum/1 -> [VINP_EPBErrSta_enum]
  VINP_CANMsgValidEPB1_flg/1 -> Logical Operator8/1
  VDDM_EPB1RCErr_flg/1 -> [VDDM_EPB1RCErr_flg]
  VDDM_EPB1CSErr_flg/1 -> [VDDM_EPB1CSErr_flg]
  Logical Operator8/1 -> [VDDM_EPB1NoCom_flg]
  [VPMM_DrivetrainSelect_enum] -> MCU_DDM/20(VPMM_DrivetrainSelect_enum)
  MCU_DDM/3(VDDM_FrMCUTqErrCFS_flg) -> [VDDM_FrMCUTqErrCFS_flg]
  MCU_DDM/4(VDDM_RrMCUTqErrCFS_flg) -> [VDDM_RrMCUTqErrCFS_flg]
  [task_time_s] -> APS_DDM/8(task_time_s)
  [VDDM_ClearZevDTCcmd_flg] -> APS_DDM/9(DTC_clear_request)
  [VDHP_EAPS1BAD_flg] -> APS_DDM/10(VDHP_EAPS1BAD_flg)
  [VDHP_EAPS2BAD_flg] -> APS_DDM/11(VDHP_EAPS2BAD_flg)
  VDHP_EAPS2BAD_flg/1 -> [VDHP_EAPS2BAD_flg]
  VDHP_EAPS1BAD_flg/1 -> [VDHP_EAPS1BAD_flg]
  APS_DDM/6(VDDM_5vAPS1OoRCFS_flg) -> [VDDM_5vAPS1OoRCFS_flg]
  APS_DDM/7(VDDM_5vAPS2OoRCFS_flg) -> [VDDM_5vAPS2OoRCFS_flg]
  APS_DDM/10(VDDM_APSCorrErrCFS_flg) -> [VDDM_APSCorrErrCFS_flg]
  APS_DDM/8(VDDM_APS1SigOoRCFS_flg) -> [VDDM_APS1SigOoRCFS_flg]
  APS_DDM/9(VDDM_APS2SigOoRCFS_flg) -> [VDDM_APS2SigOoRCFS_flg]
  [VDDM_5vAPS2OoRCFS_flg] -> VDDM_5vAPS2OoRCFS_flg/1
  [VDDM_APS1SigOoRCFS_flg] -> VDDM_APS1SigOoRCFS_flg/1
  [VDDM_5vAPS1OoRCFS_flg] -> VDDM_5vAPS1OoRCFS_flg/1
  [VDDM_APS2SigOoRCFS_flg] -> VDDM_APS2SigOoRCFS_flg/1
  [VDDM_APSCorrErrCFS_flg] -> VDDM_APSCorrErrCFS_flg/1
  [VDDM_Shifter1NoComCFS_flg] -> VDDM_Shifter1NoComCFS_flg/1
  [VDDM_Shifter1RCErrCFS_flg] -> VDDM_Shifter1RCErrCFS_flg/1
  [VDDM_Shifter1CSErrCFS_flg] -> VDDM_Shifter1CSErrCFS_flg/1
  ESC1_DDM/4(VDDM_ESC1NoComCFS_flg) -> [VDDM_ESC1NoComCFS_flg]
  ESC1_DDM/6(VDDM_ESC1CSErrCFS_flg) -> [VDDM_ESC1CSErrCFS_flg]
  ESC1_DDM/5(VDDM_ESC1RCErrCFS_flg) -> [VDDM_ESC1RCErrCFS_flg]
  [VDDM_ESC1NoComCFS_flg] -> VDDM_ESC1NoComCFS_flg/1
  [VDDM_ESC1RCErrCFS_flg] -> VDDM_ESC1RCErrCFS_flg/1
  [VDDM_ESC1CSErrCFS_flg] -> VDDM_ESC1CSErrCFS_flg/1
  ESC5_DDM/4(VDDM_ESC5NoComCFS_flg) -> [VDDM_ESC5NoComCFS_flg]
  ESC5_DDM/5(VDDM_ESC5RCErrCFS_flg) -> [VDDM_ESC5RCErrCFS_flg]
  ESC5_DDM/6(VDDM_ESC5CSErrCFS_flg) -> [VDDM_ESC5CSErrCFS_flg]
  [VDDM_ESC5NoComCFS_flg] -> VDDM_ESC5NoComCFS_flg/1
  [VDDM_ESC5RCErrCFS_flg] -> VDDM_ESC5RCErrCFS_flg/1
  [VDDM_ESC5CSErrCFS_flg] -> VDDM_ESC5CSErrCFS_flg/1
  [VDDM_EPBSigErrCFS_flg] -> VDDM_EPBSigErrCFS_flg/1
  [VDDM_EPB1NoComCFS_flg] -> VDDM_EPB1NoComCFS_flg/1
  [VDDM_EPB1RCErrCFS_flg] -> VDDM_EPB1RCErrCFS_flg/1
  [VDDM_EPB1CSErrCFS_flg] -> VDDM_EPB1CSErrCFS_flg/1
  [VDDM_EPBLockTOCFS_flg] -> VDDM_EPBLockTOCFS_flg/1
  [VDDM_EPBUnlockTOCFS_flg] -> VDDM_EPBUnlockTOCFS_flg/1
  [VDDM_FrMCUTqErrCFS_flg] -> VDDM_FrMCUTqErrCFS_flg/1
  [VDDM_RrMCUTqErrCFS_flg] -> VDDM_RrMCUTqErrCFS_flg/1
  Constant11/1 -> Switch2/1
  OR9/1 -> OR8/2
  OR7/1 -> OR3/4
  [VINP_MCUWarnF_enum] -> Equal7/1, Equal6/2
  Equal10/1 -> OR11/2
  [VINP_BMSWarn4_flg] -> OR3/1
  [VINP_BMSWarn8_flg] -> OR4/2
  Constant1/1 -> Equal1/2
  OR3/1 -> Switch6/2
  Constant17/1 -> Equal2/2
  Constant2/1 -> Equal3/1
  Constant4/1 -> Equal5/2
  Constant15/1 -> Switch6/1
  Constant7/1 -> Equal8/2
  Equal2/1 -> OR3/3
  OR6/1 -> OR5/2
  Equal1/1 -> OR5/1
  OR4/1 -> Switch1/2
  [VPMM_DrivetrainSelect_enum] -> Equal5/1
  Equal6/1 -> OR9/1
  Constant16/1 -> Switch6/3
  Equal11/1 -> OR13/1
  Constant3/1 -> Equal4/2
  Equal8/1 -> OR11/1
  Constant5/1 -> Equal6/1
  OR8/1 -> OR7/2
  Equal9/1 -> OR13/2
  Equal5/1 -> OR8/1
  [VINP_MCUWarnR_enum] -> Equal4/1, Equal3/2
  OR10/1 -> Switch2/2
  Equal4/1 -> OR6/2
  OR5/1 -> OR7/1
  [VINP_BMSWarn7_flg] -> OR4/1
  Constant9/1 -> Equal10/2
  [VINP_BMSWarn5_flg] -> OR3/2
  [VPMM_DrivetrainSelect_enum] -> Equal11/1
  OR11/1 -> OR12/1
  Constant10/1 -> Equal9/2
  [VPMM_DrivetrainSelect_enum] -> Equal8/1
  Switch6/1 -> Switch2/3
  Constant8/1 -> Equal11/2
  [VINP_MCUWarnF_enum] -> Equal9/1
  Switch1/1 -> [VDDM_VehMalfunLevelTmp_enum]  "VDDM_VehMalfunLevelTmp_enum"
  Switch2/1 -> Switch1/3
  Equal3/1 -> OR6/1
  OR13/1 -> OR12/2
  Constant6/1 -> Equal7/2
  [VINP_DCDCFaultSta_enum] -> Equal2/1
  Constant12/1 -> Switch1/1
  Equal7/1 -> OR9/2
  [VPMM_DrivetrainSelect_enum] -> Equal1/1
  [VINP_MCUWarnR_enum] -> Equal10/1
  OR/1 -> [VDDM_EDriveSysErrTQD_flg]  "VDDM_EDriveSysErrTQD_flg"
  [VDDM_VCUEPBErr_flg] -> OR/4
  APS_DDM/3(VDDM_APSCorrErrDTC_raw32) -> [VDDM_APSCorrErrDTC_raw32]
  APS_DDM/2(VDDM_APS2SigOoRDTC_raw32) -> [VDDM_APS2SigOoRDTC_raw32]
  APS_DDM/1(VDDM_APS1SigOoRDTC_raw32) -> [VDDM_APS1SigOoRDTC_raw32]
  [VDDM_APS1SigOoRDTC_raw32] -> VDDM_APS1SigOoRDTC_raw32/1
  [VDDM_APS2SigOoRDTC_raw32] -> VDDM_APS2SigOoRDTC_raw32/1
  [VDDM_APSCorrErrDTC_raw32] -> VDDM_APSCorrErrDTC_raw32/1
  MCU1_DDM/1(VDDM_MCUF1NoComDTC_raw32) -> [VDDM_MCUF1NoComDTC_raw32]
  MCU1_DDM/2(VDDM_MCUR1NoComDTC_raw32) -> [VDDM_MCUR1NoComDTC_raw32]
  [VDDM_MCUF1NoComDTC_raw32] -> VDDM_MCUF1NoComDTC_raw32/1
  [VDDM_MCUR1NoComDTC_raw32] -> VDDM_MCUR1NoComDTC_raw32/1
  Shifter1_DDM/1(VDDM_Shifter1NoComDTC_raw32) -> [VDDM_Shifter1NoComDTC_raw32]
  ESC1_DDM/1(VDDM_ESC1NoComDTC_raw32) -> [VDDM_ESC1NoComDTC_raw32]
  ESC5_DDM/1(VDDM_ESC5NoComDTC_raw32) -> [VDDM_ESC5NoComDTC_raw32]
  [VDDM_Shifter1NoComDTC_raw32] -> VDDM_Shifter1NoComDTC_raw32/1
  [VDDM_ESC1NoComDTC_raw32] -> VDDM_ESC1NoComDTC_raw32/1
  [VDDM_ESC5NoComDTC_raw32] -> VDDM_ESC5NoComDTC_raw32/1
  MCU1_DDM/3(VDDM_MCUF1RCErrDTC_raw32) -> [VDDM_MCUF1RCErrDTC_raw32]
  MCU1_DDM/4(VDDM_MCUR1RCErrDTC_raw32) -> [VDDM_MCUR1RCErrDTC_raw32]
  MCU1_DDM/5(VDDM_MCUF1CSErrDTC_raw32) -> [VDDM_MCUF1CSErrDTC_raw32]
  MCU1_DDM/6(VDDM_MCUR1CSErrDTC_raw32) -> [VDDM_MCUR1CSErrDTC_raw32]
  [VDDM_MCUF1RCErrDTC_raw32] -> VDDM_MCUF1RCErrDTC_raw32/1
  [VDDM_MCUR1RCErrDTC_raw32] -> VDDM_MCUR1RCErrDTC_raw32/1
  [VDDM_MCUF1CSErrDTC_raw32] -> VDDM_MCUF1CSErrDTC_raw32/1
  [VDDM_MCUR1CSErrDTC_raw32] -> VDDM_MCUR1CSErrDTC_raw32/1
  Shifter1_DDM/2(VDDM_Shifter1RCErrDTC_raw32) -> [VDDM_Shifter1RCErrDTC_raw32]
  Shifter1_DDM/3(VDDM_Shifter1CSErrDTC_raw32) -> [VDDM_Shifter1CSErrDTC_raw32]
  ESC1_DDM/2(VDDM_ESC1RCErrDTC_raw32) -> [VDDM_ESC1RCErrDTC_raw32]
  [VDDM_Shifter1RCErrDTC_raw32] -> VDDM_Shifter1RCErrDTC_raw32/1
  [VDDM_Shifter1CSErrDTC_raw32] -> VDDM_Shifter1CSErrDTC_raw32/1
  [VDDM_ESC1RCErrDTC_raw32] -> VDDM_ESC1RCErrDTC_raw32/1
  ESC1_DDM/3(VDDM_ESC1CSErrDTC_raw32) -> [VDDM_ESC1CSErrDTC_raw32]
  ESC5_DDM/2(VDDM_ESC5RCErrDTC_raw32) -> [VDDM_ESC5RCErrDTC_raw32]
  ESC5_DDM/3(VDDM_ESC5CSErrDTC_raw32) -> [VDDM_ESC5CSErrDTC_raw32]
  [VDDM_ESC1CSErrDTC_raw32] -> VDDM_ESC1CSErrDTC_raw32/1
  [VDDM_ESC5RCErrDTC_raw32] -> VDDM_ESC5RCErrDTC_raw32/1
  [VDDM_ESC5CSErrDTC_raw32] -> VDDM_ESC5CSErrDTC_raw32/1
  MCU_DDM/2(VDDM_RrMCUTqErrDTC_raw32) -> [VDDM_RrMCUTqErrDTC_raw32]
  MCU_DDM/1(VDDM_FrMCUTqErrDTC_raw32) -> [VDDM_FrMCUTqErrDTC_raw32]
  [VDDM_FrMCUTqErrDTC_raw32] -> VDDM_FrMCUTqErrDTC_raw32/1
  [VDDM_RrMCUTqErrDTC_raw32] -> VDDM_RrMCUTqErrDTC_raw32/1
  APS_DDM/4(VDDM_5vAPS1OoRDTC_raw32) -> [VDDM_5vAPS1OoRDTC_raw32]
  APS_DDM/5(VDDM_5vAPS2OoRDTC_raw32) -> [VDDM_5vAPS2OoRDTC_raw32]
  [VDDM_5vAPS1OoRDTC_raw32] -> VDDM_5vAPS1OoRDTC_raw32/1
  [VDDM_5vAPS2OoRDTC_raw32] -> VDDM_5vAPS2OoRDTC_raw32/1
  [VDDM_EDriveSysErrTQD_flg] -> VDDM_EDriveSysErrTQD_flg/1
  [VDDM_EDriveSysErrShifterErr_flg] -> VDDM_EDriveSysErrShifterErr_flg/1
  [VDDM_EngagePFail_flg] -> VDDM_EngagePFail_flg/1
  EPB/2(VDDM_EPBUnlockTODTC_raw32) -> [VDDM_EPBUnlockTODTC_raw32]
  EPB/1(VDDM_EPBLockTODTC_raw32) -> [VDDM_EPBLockTODTC_raw32]
  EPB/5(VDDM_EPB1NoComDTC_raw32) -> [VDDM_EPB1NoComDTC_raw32]
  EPB/6(VDDM_EPB1RCErrDTC_raw32) -> [VDDM_EPB1RCErrDTC_raw32]
  EPB/8(VDDM_EPBSigErrDTC_raw32) -> [VDDM_EPBSigErrDTC_raw32]
  EPB/7(VDDM_EPB1CSErrDTC_raw32) -> [VDDM_EPB1CSErrDTC_raw32]
  [VDDM_EPBLockTODTC_raw32] -> VDDM_EPBLockTODTC_raw32/1
  [VDDM_EPBUnlockTODTC_raw32] -> VDDM_EPBUnlockTODTC_raw32/1
  [VDDM_EPB1NoComDTC_raw32] -> VDDM_EPB1NoComDTC_raw32/1
  [VDDM_EPB1RCErrDTC_raw32] -> VDDM_EPB1RCErrDTC_raw32/1
  [VDDM_EPB1CSErrDTC_raw32] -> VDDM_EPB1CSErrDTC_raw32/1
  [VDDM_EPBSigErrDTC_raw32] -> VDDM_EPBSigErrDTC_raw32/1
  [VDDM_DisengagePFail_flg] -> VDDM_DisengagePFail_flg/1
  [VINP_HVBattSOC_pct] -> Terminator/1
  [VDDM_AuxBattVolV_V] -> Terminator1/1
  Constant13/1 -> Equal12/2
  Equal12/1 -> Logical Operator2/2
  [VTQD_GearActualPosn_enum] -> Equal12/1
  Logical Operator2/1 -> OR1/6
  [VDDM_VCUEPBErr_flg] -> Logical Operator2/1
  OR12/1 -> OR10/2
  [VINP_BMSWarn6_flg] -> OR10/1
  From112/1 -> OR15/1
  VDDM_C3BMS1LCCFS_flg/1 -> [VDDM_C3BMS1LCCFS_flg]
  From176/1 -> OR15/2
  Shifter1_DDM/7(VDDM_Shifter1Err_flg) -> [VDDM_Shifter1Err_flg]
  [VDDM_Shifter1Err_flg] -> VDDM_Shifter1Err_flg/1
  EPB/13(VDDM_EPB1Err_flg) -> [VDDM_EPB1Err_flg]
  [VDDM_EPB1Err_flg] -> VDDM_EPB1Err_flg/1
  ESC1_DDM/7(VDDM_ESC1Err_flg) -> [VDDM_ESC1Err_flg]
  ESC5_DDM/7(VDDM_ESC5Err_flg) -> [VDDM_ESC5Err_flg]
  [VDDM_ESC5Err_flg] -> VDDM_ESC5Err_flg/1
  [VDDM_ESC1Err_flg] -> VDDM_ESC1Err_flg/1
  [VVMC_APSActive_flg] -> Logical Operator11/2
  [VDDM_VCURAPSErrLv2_flg] -> Logical Operator11/1
  Logical Operator11/1 -> OR1/7
  VVMC_APSActive_flg/1 -> [VVMC_APSActive_flg]
  VDDM_VCURAPSErrLv2_flg/1 -> [VDDM_VCURAPSErrLv2_flg]
  OR1/1 -> Switch/1
  Constant/1 -> Switch/2
  Constant21/1 -> Switch/3
  VDDM_ClearZevDTCcmd_flg/1 -> [VDDM_ClearZevDTCcmd_flg]
  [VTQR_FrTqZeroTrans_enum] -> MCU_DDM/21(VTQR_FrTqZeroTrans_enum)
  [VTQR_RrTqZeroTrans_enum] -> MCU_DDM/22(VTQR_RrTqZeroTrans_enum)
  Regen_fail_DDM/2(VDDM_RegenErrCFS_flg) -> [VDDM_RegenErrCFS_flg]
  [DTC_clear_request] -> Regen_fail_DDM/4(DTC_clear_request)
  [VDDM_LimpHomeAct_flg] -> Regen_fail_DDM/3(VDDM_LimpHomeAct_flg)
  [task_time_s] -> Regen_fail_DDM/1(task_time_s)
  [VPMM_SysPwrSta_enum] -> Regen_fail_DDM/2(VPMM_SysPwrSta_enum)
  Regen_fail_DDM/1(VDDM_RegenErrDTC_raw32) -> [VDDM_RegenErrDTC_raw32]
  VDDM_LimpHomeAct_flg/1 -> [VDDM_LimpHomeAct_flg]
  Logical Operator12/1 -> Logical Operator14/1
  Delay3/1 -> Logical Operator15/2
  [VDDM_EPBUnlockTOCFS_flg] -> OR14/1
  Switch4/1 -> [VDDM_DisengagePFail_flg]  "VDDM_DisengagePFail_flg"
  Delay/1 -> Logical Operator14/2
  Logical Operator7/1 -> SR_Latch1/1
  Logical Operator14/1 -> SR_Latch1/2
  [VDDM_DisengagePFail_flg] -> Delay/1
  Logical Operator10/1 -> SR_Latch2/1
  Constant22/1 -> Switch3/2
  Switch3/1 -> [VDDM_EngagePFail_flg]  "VDDM_EngagePFail_flg"
  Constant24/1 -> Switch4/2
  OR2/1 -> Switch3/1
  Equal15/1 -> Logical Operator10/2
  OR14/1 -> Switch4/1
  Constant23/1 -> Switch3/3
  Constant19/1 -> Equal14/2
  [VDDM_EPBLockTOCFS_flg] -> OR2/2
  Constant88/1 -> Equal/2
  [VDDM_VCUEPBErr_flg] -> Logical Operator13/1
  [VTQD_GearActualPosn_enum] -> Equal13/1
  [VTQD_GearActualPosn_enum] -> Delay2/1
  Logical Operator13/1 -> Logical Operator15/1
  Constant25/1 -> Switch4/3
  Equal14/1 -> Logical Operator10/1
  [VDDM_VCUEPBErr_flg] -> Logical Operator12/1
  [VDDM_VCURAPSErrLv2_flg] -> Logical Operator6/1
  SR_Latch1/1 -> OR2/3
  Logical Operator6/1 -> OR2/1
  Constant20/1 -> Equal16/2
  [VDDM_VCUEPBErr_flg] -> Logical Operator10/4
  Delay1/1 -> Equal/1
  Constant18/1 -> Equal15/1
  Delay2/1 -> Equal14/1
  Constant14/1 -> Equal13/2
  [VVMC_APSActive_flg] -> Logical Operator6/2
  Equal13/1 -> Logical Operator7/2
  [VDDM_EPB1RCErrCFS_flg] -> Logical Operator9/3
  Logical Operator9/1 -> [VDDM_VCUEPBErr_flg]  "VDDM_VCUEPBErr_flg"
  [VDDM_EPB1CSErrCFS_flg] -> Logical Operator9/4
  Equal16/1 -> Logical Operator10/3
  [VDDM_EPB1NoComCFS_flg] -> Logical Operator9/2
  Equal/1 -> Logical Operator7/1
  SR_Latch2/1 -> OR14/2
  [VDDM_VCUEPBErr_flg] -> Logical Operator7/3
  [VDDM_EPBSigErrCFS_flg] -> Logical Operator9/1
  [VTQD_GearActualPosn_enum] -> Equal16/1, Equal15/2
  Logical Operator15/1 -> SR_Latch2/2
  [VTQD_GearActualPosn_enum] -> Delay1/1
  [VDDM_EngagePFail_flg] -> Delay3/1
  [VDDM_RegenErrCFS_flg] -> VDDM_RegenErrCFS_flg/1
  [VDDM_RegenErrDTC_raw32] -> VDDM_RegenErrDTC_raw32/1
  VTQR_FrTqZeroTrans_enum/1 -> [VTQR_FrTqZeroTrans_enum]
  VTQR_RrTqZeroTrans_enum/1 -> [VTQR_RrTqZeroTrans_enum]
  MCU1_DDM/13(VDDM_MCUF1Err_flg) -> [VDDM_MCUF1Err_flg]
  MCU1_DDM/14(VDDM_MCUR1Err_flg) -> [VDDM_MCUR1Err_flg]
  [VDDM_MCUF1Err_flg] -> VDDM_MCUF1Err_flg/1
  [VDDM_MCUR1Err_flg] -> VDDM_MCUR1Err_flg/1
